simulink library "ScalarChimeControlLibBtc"  (R2022b)
settings: Solver=VariableStepAuto  StartTime=0.0  StopTime=10.0  RelTol=1e-3
libraries: ChimeControlLibBtc x1, HandyTextFile x1, RgainzBtc x1, simulink x1
settings Model: Creator=kl13806  LastModifiedBy=kl13806
settings SolverCC: AlgebraicLoopSolver=TrustRegion
settings DebuggingCC: UnconnectedInputMsg=warning  UnconnectedOutputMsg=warning  UnconnectedLineMsg=warning  SFMachineParentedDataDiag=warning
settings ModelReferenceCC: EnableRefExpFcnMdlSchedulingChecks=on
settings RTWCC: DLArmComputeVersion=19.05

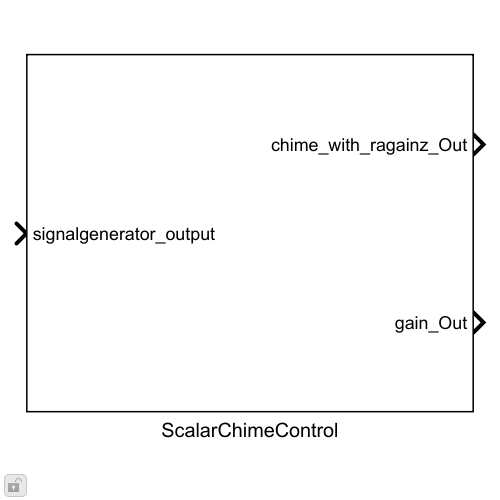
[thumbnail: Simulink's stored preview of the top-level diagram]
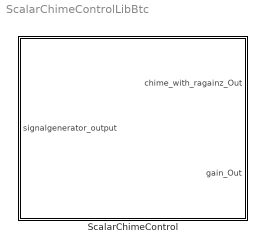
== system ScalarChimeControlLibBtc ==
  ScalarChimeControl : Subsystem  mask{Config=[]}
      mask prompts: Config "ScalarChimeControlConfig"
      mask init:
      | blkh=gcbh;
      | Config=BTConfig.Assert(blkh,Config);
      | 
      | Config.Validate();

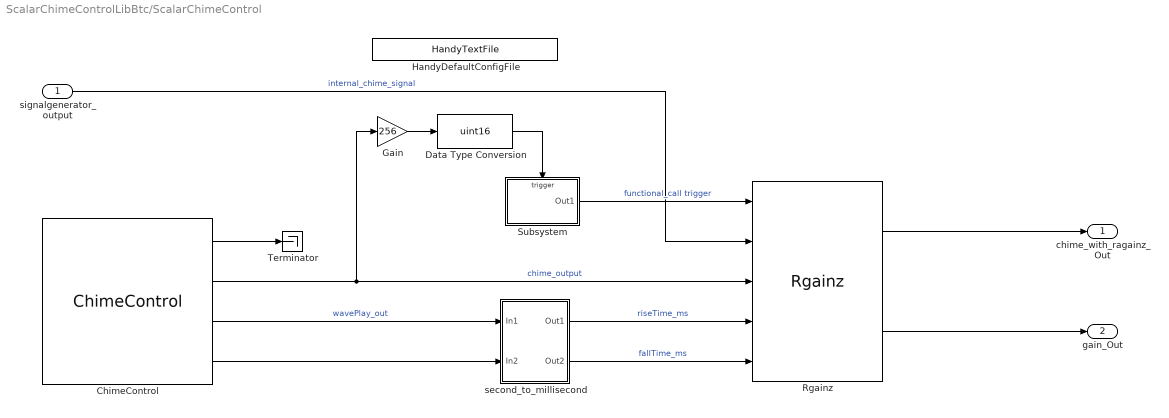
== system ScalarChimeControlLibBtc/ScalarChimeControl ==
  signalgenerator_output : Inport
  ChimeControl : ChimeControlLibBtc/ChimeControl  Config=Config  FeatureName=Control
      settings: SourceProductName=Bose Blocklib
  Data Type Conversion : DataTypeConversion  OutDataTypeStr=uint16  SaturateOnIntegerOverflow=off  RndMeth=Floor
  Gain : Gain  Gain=256
  HandyDefaultConfigFile : HandyTextFile/HandyTextFile  TemplateSource=Config  FileSuffix=Init  OpenDialogOnLoad=off  UseThisBlockName=off  TheDefaultText=|  ShowInLibBrowser=on
      | % $(FILENAME) Setup model parameters for each "Init" callback (e.g. update diagram)
      | sample_rate_in_hertz = 44100;
      | frame_size = 32;
      | sysin_channel_count = 2;
  Rgainz : RgainzBtc/Rgainz  Config=Config.Rgainz
      settings: SourceProductName=Bose Blocklib
  Subsystem : Subsystem
  Terminator : Terminator
  second_to_millisecond : Subsystem
  chime_with_ragainz_Out : Outport  VectorParamsAs1DForOutWhenUnconnected=off
  gain_Out : Outport  Port=2  VectorParamsAs1DForOutWhenUnconnected=off
  wires:
  ChimeControl/1 -> Terminator/1
  signalgenerator_output/1 -> Rgainz/2  "internal_chime_signal"
  Rgainz/1 -> chime_with_ragainz_Out/1
  Rgainz/2 -> gain_Out/1
  ChimeControl/2 -> Gain/1, Rgainz/3  "chime_output"
  Data Type Conversion/1 -> Subsystem/Trigger
  Subsystem/1(Out1) -> Rgainz/1  "functional_call trigger"
  second_to_millisecond/1(Out1) -> Rgainz/4  "riseTime_ms"
  second_to_millisecond/2(Out2) -> Rgainz/5  "fallTime_ms"
  ChimeControl/3 -> second_to_millisecond/1(In1)  "wavePlay_out"
  ChimeControl/4 -> second_to_millisecond/2(In2)
  Gain/1 -> Data Type Conversion/1

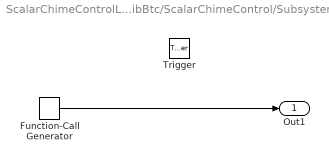
== system ScalarChimeControlLibBtc/ScalarChimeControl/Subsystem ==
  Trigger : TriggerPort  TriggerType=either  VariantControl=Variant  PortDimensions=1
  Function-Call Generator : simulink/Ports & Subsystems/Function-Call Generator  sample_time=-1  numberOfIterations=1  DisallowWideOutput=off
  Out1 : Outport  VectorParamsAs1DForOutWhenUnconnected=off
  wires:
  Function-Call Generator/1 -> Out1/1

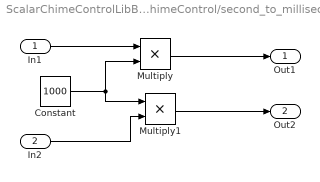
== system ScalarChimeControlLibBtc/ScalarChimeControl/second_to_millisecond ==
  In1 : Inport
  In2 : Inport  Port=2
  Constant : Constant  Value=1000
  Multiply : Product
  Multiply1 : Product
  Out1 : Outport  VectorParamsAs1DForOutWhenUnconnected=off
  Out2 : Outport  Port=2  VectorParamsAs1DForOutWhenUnconnected=off
  wires:
  Multiply1/1 -> Out2/1
  Multiply/1 -> Out1/1
  Constant/1 -> Multiply1/1, Multiply/2
  In2/1 -> Multiply1/2
  In1/1 -> Multiply/1
